simulink subsystem "RCS_THRUSTER"  (R2025b)
settings: Solver=VariableStepAuto  StartTime=0.0  StopTime=10.0  RelTol=1e-3
model mask{rcsIsp=0, rcsMaxMdot=0}
  mask prompts: rcsIsp "Specific impulse [ms-1]"; rcsMaxMdot "Maximum mass flow rate [kgs-1]"
settings Model: Creator=antoniohernandez-rodiciomateos  LastModifiedBy=antoniohernandez-rodiciomateos

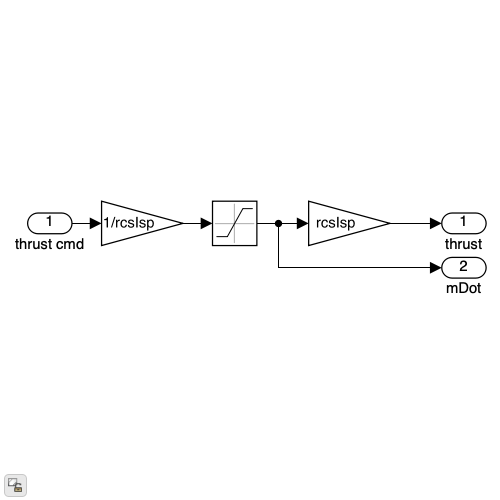
[thumbnail: Simulink's stored preview of the top-level diagram]
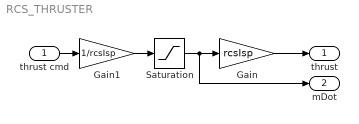
== system RCS_THRUSTER ==
  thrust cmd : Inport  OutDataTypeStr=double  PortDimensions=[1 1]
  Gain : Gain  Gain=rcsIsp
  Gain1 : Gain  Gain=1/rcsIsp
  Saturation : Saturate  UpperLimit=rcsMaxMdot  LowerLimit=0
  thrust : Outport  OutDataTypeStr=double  PortDimensions=[1 1]
  mDot : Outport  Port=2  OutDataTypeStr=double  PortDimensions=[1 1]
  wires:
  Saturation/1 -> mDot/1, Gain/1
  Gain/1 -> thrust/1
  Gain1/1 -> Saturation/1
  thrust cmd/1 -> Gain1/1
